simulink model "model_mimo"  (Simulink 7.4)
settings: Solver=ode3  StartTime=0.0  StopTime=T-Ts  FixedStep=Ts  RelTol=1e-3
values from neighbouring files (symbols this model uses):
  sys = sys(1:2,1:2)    [main_mimo.m]    (also in main_siso.m = sys(1,2))
  Ts = 1/Fs    [definitions.m]    (also in main_hess.m = 0.05; main_mimo.m = 0.1; main_rider.m = 0.02; main_rider_time.m = 0.02)
libraries: cstblocks x1
settings Model: Creator=Peter  LastModifiedBy=Peter
settings DataIOCC: SaveOutput=off  SaveTime=off

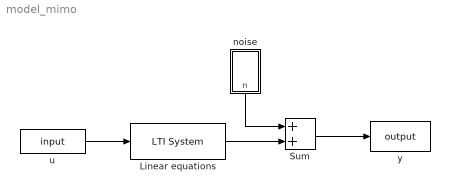
== system model_mimo ==
  Linear equations : cstblocks/LTI System  SystemSampleTime=-1  sys=sys;  IC=zeros(4,1);
  Sum : Sum  OutDataType=sfix(16)  OutScaling=2^0  SaturateOnIntegerOverflow=on  InputSameDT=on  OutDataTypeStr=Inherit: Same as first input
  noise : Subsystem
  u : FromWorkspace  VariableName=input  SampleTime=Ts
  y : ToWorkspace  VariableName=output  SampleTime=Ts  SaveFormat=Structure With Time
      settings: Description=output
  wires:
  Linear equations/1 -> Sum/2
  Sum/1 -> y/1
  noise/1(n) -> Sum/1
  u/1 -> Linear equations/1

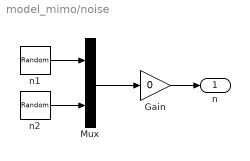
== system model_mimo/noise ==
  Gain : Gain  Gain=0  ParameterDataType=fixdt(1, 16)  ParameterScaling=2^0  OutDataType=fixdt(1, 16)  OutScaling=2^0
  Mux : Mux  Inputs=2
  n1 : RandomNumber  Seed=61  SampleTime=Ts
  n2 : RandomNumber  Seed=61  SampleTime=Ts
  n : Outport  OutDataType=fixdt(1, 16)  OutScaling=2^0
  wires:
  Mux/1 -> Gain/1
  n1/1 -> Mux/1
  n2/1 -> Mux/2
  Gain/1 -> n/1
